simulink model "motor_eq_mk1"  (R2015b)
settings: Solver=ode4  StartTime=0.0  StopTime=1  FixedStep=0.0002  RelTol=1e-3
values from neighbouring files (symbols this model uses):
  Beq = 0.015    [parameter.m]
  Jeq = 9.76e-5    (= 9.76e-05)    [parameter.m]
  Ka = eta_g * Kg * eta_m * kt / Jeq    (= 3420.59016393)    [parameter.m]
  Kb = km * Kg    (= 0.5376)    [parameter.m]
  Lm = 0.18e-3    (= 0.00018)    [parameter.m]
  Rm = 2.6    [parameter.m]
settings Model: ExtModeTrigDuration=10000  Creator=flynng  LastModifiedBy=flynng
settings SolverCC: PositivePriorityOrder=on
settings RTWCC: SystemTargetFile=quarc_win64.tlc  TemplateMakefile=quarc_default_tmf  Description=QUARC Win64 Target
settings STFCustomTargetCC: TargetPreCompLibLocation=C:\ProgramData\QUARC\lib\2015b\win64\release  GeneratePreprocessorConditionals=Use local settings  CPPClassGenCompliant=off
settings GRTTargetCC: TargetPreCompLibLocation=C:\ProgramData\QUARC\lib\2015b\win64\release  ParMdlRefBuildCompliant=off  CompOptLevelCompliant=off  CombineOutputUpdateFcns=off  MatFileLogging=off  CPPClassGenCompliant=off  GRTInterface=on  UseToolchainInfoCompliant=off  ExtMode=on  ExtModeMexFile=quarc_comm

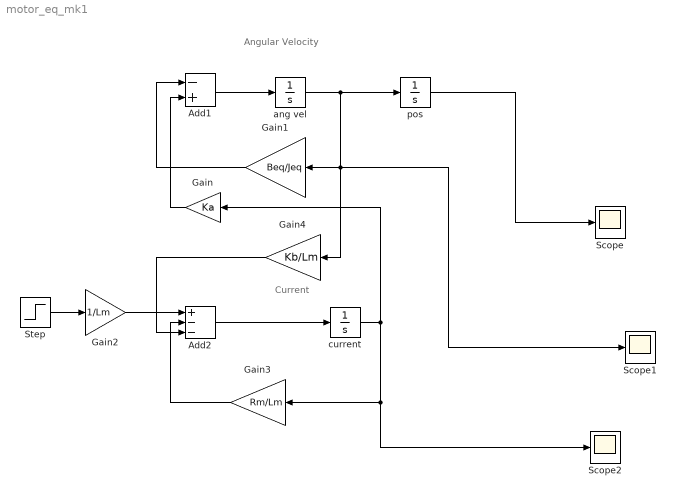
== system motor_eq_mk1 ==
  note: Current
  note: Angular Velocity
  Add1 : Sum  Inputs=-+
  Add2 : Sum  Inputs=+--
  Gain : Gain  Gain=Ka
  Gain1 : Gain  Gain=Beq/Jeq
  Gain2 : Gain  Gain=1/Lm
  Gain3 : Gain  Gain=Rm/Lm
  Gain4 : Gain  Gain=Kb/Lm
  Scope : Scope
  Scope1 : Scope
  Scope2 : Scope
  Step : Step  Time=0  SampleTime=0
  ang vel : Integrator
  current : Integrator
  pos : Integrator
  wires:
  Add2/1 -> current/1
  Gain/1 -> Add1/2
  Step/1 -> Gain2/1
  Gain2/1 -> Add2/1
  current/1 -> Gain/1, Scope2/1, Gain3/1
  Gain3/1 -> Add2/2
  Gain4/1 -> Add2/3
  Add1/1 -> ang vel/1
  ang vel/1 -> Scope1/1, Gain4/1, Gain1/1, pos/1
  Gain1/1 -> Add1/1
  pos/1 -> Scope/1
